simulink model "Experiment_Setup_Simulation"  (R2018b)
settings: Solver=FixedStepDiscrete  StartTime=0.0  StopTime=inf  FixedStep=0.02  RelTol=1e-3
libraries: simulink x4
settings Model: EnablePacing=on  PacingRate=2  Creator=Daniele Nava  LastModifiedBy=Daniele Nava

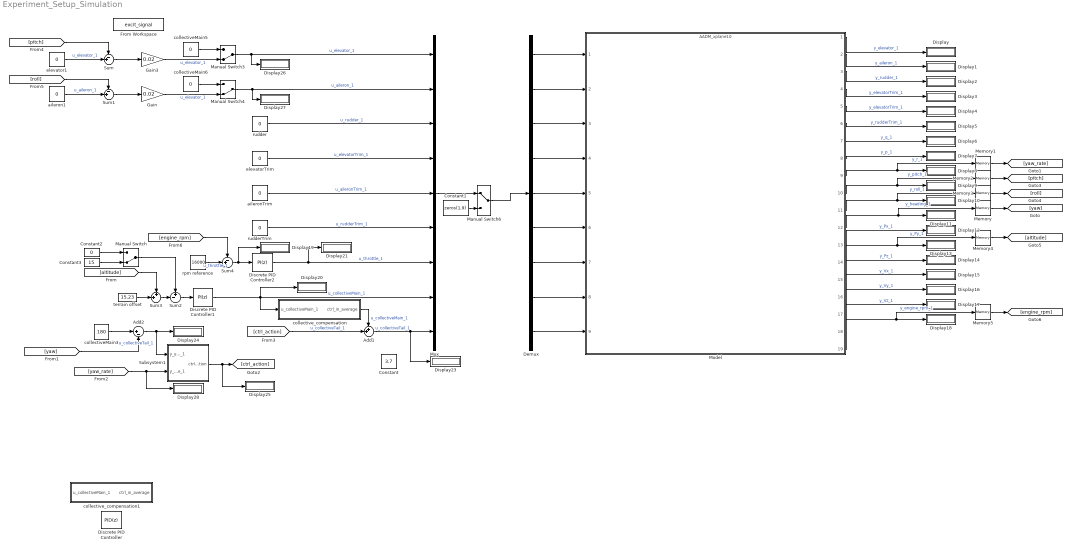
== system Experiment_Setup_Simulation ==
  Add1 : Sum  Inputs=++|
  Add2 : Sum  Inputs=|+-
  Constant : Constant  Value=3.7
  Constant1 : Constant  Value=zeros(1,9)
  Constant2 : Constant  Value=0
  Constant3 : Constant  Value=15
  Demux : Demux  Outputs=9
  Discrete PID Controller : simulink/Continuous/PID Controller  Controller=PID  Form=Parallel  TimeDomain=Discrete-time  SampleTime=-1  IntegratorMethod=Forward Euler  FilterMethod=Forward Euler  ControllerParametersSource=internal  P=1  I=1  D=0  UseFilter=on  N=100  TunerSelectOption=Transfer Function Based (PID Tuner App)  InitialConditionSource=internal  InitialConditionForIntegrator=0  InitialConditionForFilter=0  DifferentiatorICPrevScaledInput=0  ExternalReset=none  TrackingMode=off  Kt=1  LimitOutput=off  UpperSaturationLimit=inf  LowerSaturationLimit=-inf  LinearizeAsGain=off  AntiWindupMode=none  Kb=1  POutMin=[]  POutMax=[]  IOutMin=[]  IOutMax=[]  DOutMin=[]  DOutMax=[]  NOutMin=[]  NOutMax=[]  SumOutMin=[]  SumOutMax=[]  SaturationOutMin=[]  SaturationOutMax=[]  PParamMin=[]  PParamMax=[]  IParamMin=[]  IParamMax=[]  DParamMin=[]  DParamMax=[]  NParamMin=[]  NParamMax=[]  KbParamMin=[]  KbParamMax=[]  KtParamMin=[]  KtParamMax=[]  KbOutMin=[]  KbOutMax=[]  KtOutMin=[]  KtOutMax=[]  IntegratorOutMin=[]  IntegratorOutMax=[]  FilterOutMin=[]  FilterOutMax=[]  SumI1OutMin=[]  SumI1OutMax=[]  SumI2OutMin=[]  SumI2OutMax=[]  SumI3OutMin=[]  SumI3OutMax=[]  SumI4OutMin=[]  SumI4OutMax=[]  SumDOutMin=[]  SumDOutMax=[]  DifferentiatorOutMin=[]  DifferentiatorOutMax=[]  FilterDiffOutCoefMin=[]  FilterDiffOutCoefMax=[]  ReciprocalOutMin=[]  ReciprocalOutMax=[]  SumDenOutMin=[]  SumDenOutMax=[]  SumNumOutMin=[]  SumNumOutMax=[]  DivideOutMin=[]  DivideOutMax=[]  IntegratorContinuousStateAttributes=''  IntegratorStateMustResolveToSignalObject=off  IntegratorRTWStateStorageClass=Auto  FilterContinuousStateAttributes=''  FilterStateMustResolveToSignalObject=off  FilterRTWStateStorageClass=Auto  ParallelPVariant=InternalParameters  IdealPVariant=Disabled  IVariant=InternalParameters  DVariant=InternalParameters  IntegratorVariant=Discrete  SatVariant=Disabled  AWVariant=Passthrough  PCopyVariant=Disabled  TRVariant=Disabled  FdbkBlocksVariant=Forward  IdealPFdbkVariant=Disabled  SatFdbkVariant=Disabled  DerivativeFilterVariant=ForwardEulerFilter  NVariant=InternalParameters  NCopyVariant=Disabled  FilterICVariant=InternalICsFilter  IntegratorICVariant=InternalICs  ExternalResetVariant=Disabled  TRSumVariant=Passthrough  SumFdbkVariant=Disabled  SumVariant=Sum_PID
  Discrete PID Controller1 : simulink/Continuous/PID Controller  Controller=PI  Form=Parallel  TimeDomain=Discrete-time  SampleTime=-1  IntegratorMethod=Forward Euler  FilterMethod=Forward Euler  ControllerParametersSource=internal  P=0.5  I=0.2  D=0  UseFilter=on  N=100  TunerSelectOption=Transfer Function Based (PID Tuner App)  InitialConditionSource=internal  InitialConditionForIntegrator=0  InitialConditionForFilter=0  DifferentiatorICPrevScaledInput=0  ExternalReset=none  TrackingMode=off  Kt=1  LimitOutput=off  UpperSaturationLimit=inf  LowerSaturationLimit=-inf  LinearizeAsGain=off  AntiWindupMode=none  Kb=1  POutMin=[]  POutMax=[]  IOutMin=[]  IOutMax=[]  DOutMin=[]  DOutMax=[]  NOutMin=[]  NOutMax=[]  SumOutMin=[]  SumOutMax=[]  SaturationOutMin=[]  SaturationOutMax=[]  PParamMin=[]  PParamMax=[]  IParamMin=[]  IParamMax=[]  DParamMin=[]  DParamMax=[]  NParamMin=[]  NParamMax=[]  KbParamMin=[]  KbParamMax=[]  KtParamMin=[]  KtParamMax=[]  KbOutMin=[]  KbOutMax=[]  KtOutMin=[]  KtOutMax=[]  IntegratorOutMin=[]  IntegratorOutMax=[]  FilterOutMin=[]  FilterOutMax=[]  SumI1OutMin=[]  SumI1OutMax=[]  SumI2OutMin=[]  SumI2OutMax=[]  SumI3OutMin=[]  SumI3OutMax=[]  SumI4OutMin=[]  SumI4OutMax=[]  SumDOutMin=[]  SumDOutMax=[]  DifferentiatorOutMin=[]  DifferentiatorOutMax=[]  FilterDiffOutCoefMin=[]  FilterDiffOutCoefMax=[]  ReciprocalOutMin=[]  ReciprocalOutMax=[]  SumDenOutMin=[]  SumDenOutMax=[]  SumNumOutMin=[]  SumNumOutMax=[]  DivideOutMin=[]  DivideOutMax=[]  IntegratorContinuousStateAttributes=''  IntegratorStateMustResolveToSignalObject=off  IntegratorRTWStateStorageClass=Auto  FilterContinuousStateAttributes=''  FilterStateMustResolveToSignalObject=off  FilterRTWStateStorageClass=Auto  ParallelPVariant=InternalParameters  IdealPVariant=Disabled  IVariant=InternalParameters  DVariant=Disabled  IntegratorVariant=Discrete  SatVariant=Disabled  AWVariant=Passthrough  PCopyVariant=Disabled  TRVariant=Disabled  FdbkBlocksVariant=Forward  IdealPFdbkVariant=Disabled  SatFdbkVariant=Disabled  DerivativeFilterVariant=Disabled  NVariant=Disabled  NCopyVariant=Disabled_SignalSpec  FilterICVariant=Disabled  IntegratorICVariant=InternalICs  ExternalResetVariant=Disabled  TRSumVariant=Passthrough  SumFdbkVariant=Disabled  SumVariant=Sum_PI
  Discrete PID Controller2 : simulink/Continuous/PID Controller  Controller=PI  Form=Parallel  TimeDomain=Discrete-time  SampleTime=-1  IntegratorMethod=Forward Euler  FilterMethod=Forward Euler  ControllerParametersSource=internal  P=0.5  I=0.2  D=0  UseFilter=on  N=100  TunerSelectOption=Transfer Function Based (PID Tuner App)  InitialConditionSource=internal  InitialConditionForIntegrator=0  InitialConditionForFilter=0  DifferentiatorICPrevScaledInput=0  ExternalReset=none  TrackingMode=off  Kt=1  LimitOutput=off  UpperSaturationLimit=inf  LowerSaturationLimit=-inf  LinearizeAsGain=off  AntiWindupMode=none  Kb=1  POutMin=[]  POutMax=[]  IOutMin=[]  IOutMax=[]  DOutMin=[]  DOutMax=[]  NOutMin=[]  NOutMax=[]  SumOutMin=[]  SumOutMax=[]  SaturationOutMin=[]  SaturationOutMax=[]  PParamMin=[]  PParamMax=[]  IParamMin=[]  IParamMax=[]  DParamMin=[]  DParamMax=[]  NParamMin=[]  NParamMax=[]  KbParamMin=[]  KbParamMax=[]  KtParamMin=[]  KtParamMax=[]  KbOutMin=[]  KbOutMax=[]  KtOutMin=[]  KtOutMax=[]  IntegratorOutMin=[]  IntegratorOutMax=[]  FilterOutMin=[]  FilterOutMax=[]  SumI1OutMin=[]  SumI1OutMax=[]  SumI2OutMin=[]  SumI2OutMax=[]  SumI3OutMin=[]  SumI3OutMax=[]  SumI4OutMin=[]  SumI4OutMax=[]  SumDOutMin=[]  SumDOutMax=[]  DifferentiatorOutMin=[]  DifferentiatorOutMax=[]  FilterDiffOutCoefMin=[]  FilterDiffOutCoefMax=[]  ReciprocalOutMin=[]  ReciprocalOutMax=[]  SumDenOutMin=[]  SumDenOutMax=[]  SumNumOutMin=[]  SumNumOutMax=[]  DivideOutMin=[]  DivideOutMax=[]  IntegratorContinuousStateAttributes=''  IntegratorStateMustResolveToSignalObject=off  IntegratorRTWStateStorageClass=Auto  FilterContinuousStateAttributes=''  FilterStateMustResolveToSignalObject=off  FilterRTWStateStorageClass=Auto  ParallelPVariant=InternalParameters  IdealPVariant=Disabled  IVariant=InternalParameters  DVariant=Disabled  IntegratorVariant=Discrete  SatVariant=Disabled  AWVariant=Passthrough  PCopyVariant=Disabled  TRVariant=Disabled  FdbkBlocksVariant=Forward  IdealPFdbkVariant=Disabled  SatFdbkVariant=Disabled  DerivativeFilterVariant=Disabled  NVariant=Disabled  NCopyVariant=Disabled_SignalSpec  FilterICVariant=Disabled  IntegratorICVariant=InternalICs  ExternalResetVariant=Disabled  TRSumVariant=Passthrough  SumFdbkVariant=Disabled  SumVariant=Sum_PI
  Display{,1..21,23..28} (28 alike) : Display
  From Workspace : FromWorkspace  VariableName=excit_signal  SampleTime=0
  Gain : Gain  Gain=0.02
  Gain3 : Gain  Gain=0.02
  Manual Switch : ManualSwitch  CurrentSetting=0
  Manual Switch3 : ManualSwitch  CurrentSetting=0
  Manual Switch4 : ManualSwitch  CurrentSetting=0
  Manual Switch6 : ManualSwitch
  Memory{,1..5} (6 alike) : Memory
  Model : ModelReference  ModelNameDialog=AADM_xplane10.slx  SimulationMode=Normal  ModelReferenceVersion=1.12
  Mux : Mux  Inputs=9
  Subsystem1 : Subsystem  mask{Kp=-0.8, Ki=-0.01, Kd=+0.01}
      mask prompts: Kp "Proportional"; Ki "Integral"; Kd "Derivative"
  Sum : Sum  Inputs=-+|
  Sum1 : Sum  Inputs=-+|
  Sum2 : Sum  Inputs=+-|
  Sum3 : Sum  Inputs=++|
  Sum4 : Sum  Inputs=-+|
  aileron1 : Constant  Value=0
  aileronTrim : Constant  Value=0
  collectiveMain3 : Constant  Value=180
  collectiveMain5 : Constant  Value=0
  collectiveMain6 : Constant  Value=0
  collective_compensation : Subsystem
  collective_compensation1 : Subsystem
  elevator1 : Constant  Value=0
  elevatorTrim : Constant  Value=0
  rpm reference : Constant  Value=16000
  rudder : Constant  Value=0
  rudderTrim : Constant  Value=0
  terrain offset : Constant  Value=15.23
  wires:
  elevatorTrim/1 -> Mux/4  "u_elevatorTrim_1"
  Sum/1 -> Gain3/1
  Sum1/1 -> Gain/1
  aileronTrim/1 -> Mux/5  "u_aileronTrim_1"
  rudderTrim/1 -> Mux/6  "u_rudderTrim_1"
  Discrete PID Controller2/1 -> Display21/1, Mux/7  "u_throttle_1"
  Discrete PID Controller1/1 -> Display20/1, Mux/8, collective_compensation/1(u_collectiveMain_1)  "u_collectiveMain_1"
  rudder/1 -> Mux/3  "u_rudder_1"
  collectiveMain3/1 -> Add2/1
  Add2/1 -> Subsystem1/1(y_yaw_1), Display24/1  "u_collectiveTail_1"
  [ctrl_action] -> Add1/2  "u_collectiveTail_1"
  Add1/1 -> Display23/1, Mux/9  "u_collectiveTail_1"
  [yaw] -> Add2/2
  [yaw_rate] -> Display28/1, Subsystem1/2(y_yaw_rate_1)
  Subsystem1/1(ctrl_action) -> Display25/1, [ctrl_action]
  aileron1/1 -> Sum1/2  "u_aileron_1"
  elevator1/1 -> Sum/2  "u_elevator_1"
  [roll] -> Sum1/1
  [pitch] -> Sum/1
  Manual Switch3/1 -> Mux/1, Display26/1  "u_elevator_1"
  collectiveMain5/1 -> Manual Switch3/1
  Gain3/1 -> Manual Switch3/2  "u_elevator_1"
  Gain/1 -> Manual Switch4/2  "u_elevator_1"
  collectiveMain6/1 -> Manual Switch4/1
  Manual Switch4/1 -> Mux/2, Display27/1  "u_aileron_1"
  Memory3/1 -> [roll]
  Model/3 -> Display2/1  "y_rudder_1"
  Model/15 -> Display14/1  "y_Pz_1"
  Model/6 -> Display5/1  "y_rudderTrim_1"
  Memory2/1 -> [pitch]
  Model/2 -> Display1/1  "y_aileron_1"
  Model/8 -> Display7/1  "y_p_1"
  Model/4 -> Display3/1  "y_elevatorTrim_1"
  Model/10 -> Memory2/1, Display9/1  "y_pitch_1"
  Memory/1 -> [yaw]
  Model/1 -> Display/1  "y_elevator_1"
  Model/7 -> Display6/1  "y_q_1"
  Memory1/1 -> [yaw_rate]
  Model/17 -> Display16/1  "y_Vy_1"
  Model/12 -> Memory/1, Display11/1  "y_heading_1"
  Model/16 -> Display15/1  "y_Vx_1"
  Model/13 -> Display12/1  "y_Px_1"
  Model/11 -> Memory3/1, Display10/1  "y_roll_1"
  Model/18 -> Display17/1  "y_Vz_1"
  Model/5 -> Display4/1  "y_elevatorTrim_1"
  Model/9 -> Memory1/1, Display8/1  "y_r_1"
  Demux/1 -> Model/1
  Demux/2 -> Model/2
  Demux/3 -> Model/3
  Demux/4 -> Model/4
  Demux/5 -> Model/5
  Demux/6 -> Model/6
  Demux/7 -> Model/7
  Demux/8 -> Model/8
  Demux/9 -> Model/9
  Manual Switch6/1 -> Demux/1
  Mux/1 -> Manual Switch6/1
  Constant1/1 -> Manual Switch6/2
  Model/14 -> Memory4/1, Display13/1  "y_Py_1"
  Memory4/1 -> [altitude]
  Sum2/1 -> Discrete PID Controller1/1
  Sum3/1 -> Sum2/2
  Constant2/1 -> Manual Switch/1
  Constant3/1 -> Manual Switch/2
  terrain offset/1 -> Sum3/2
  [altitude] -> Sum3/1
  Manual Switch/1 -> Sum2/1
  Memory5/1 -> [engine_rpm]
  Model/19 -> Memory5/1, Display18/1  "y_engine_rpm_1"
  [engine_rpm] -> Sum4/1
  rpm reference/1 -> Sum4/2  "u_throttle_1"
  Sum4/1 -> Discrete PID Controller2/1, Display19/1
  collective_compensation/1(ctrl_in_average) -> Add1/1  "u_collectiveMain_1"

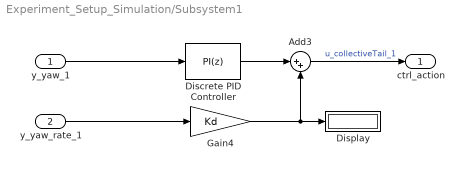
== system Experiment_Setup_Simulation/Subsystem1 ==
  y_yaw_1 : Inport
  y_yaw_rate_1 : Inport  Port=2
  Add3 : Sum  Inputs=|++
  Discrete PID Controller : simulink/Continuous/PID Controller  Controller=PI  Form=Parallel  TimeDomain=Discrete-time  SampleTime=-1  IntegratorMethod=Forward Euler  FilterMethod=Forward Euler  ControllerParametersSource=internal  P=Kp  I=Ki  D=0  UseFilter=on  N=100  TunerSelectOption=Transfer Function Based (PID Tuner App)  InitialConditionSource=internal  InitialConditionForIntegrator=0  InitialConditionForFilter=0  DifferentiatorICPrevScaledInput=0  ExternalReset=none  TrackingMode=off  Kt=1  LimitOutput=on  UpperSaturationLimit=16-8  LowerSaturationLimit=-16-8  LinearizeAsGain=off  AntiWindupMode=back-calculation  Kb=1  POutMin=[]  POutMax=[]  IOutMin=[]  IOutMax=[]  DOutMin=[]  DOutMax=[]  NOutMin=[]  NOutMax=[]  SumOutMin=[]  SumOutMax=[]  SaturationOutMin=[]  SaturationOutMax=[]  PParamMin=[]  PParamMax=[]  IParamMin=[]  IParamMax=[]  DParamMin=[]  DParamMax=[]  NParamMin=[]  NParamMax=[]  KbParamMin=[]  KbParamMax=[]  KtParamMin=[]  KtParamMax=[]  KbOutMin=[]  KbOutMax=[]  KtOutMin=[]  KtOutMax=[]  IntegratorOutMin=[]  IntegratorOutMax=[]  FilterOutMin=[]  FilterOutMax=[]  SumI1OutMin=[]  SumI1OutMax=[]  SumI2OutMin=[]  SumI2OutMax=[]  SumI3OutMin=[]  SumI3OutMax=[]  SumI4OutMin=[]  SumI4OutMax=[]  SumDOutMin=[]  SumDOutMax=[]  DifferentiatorOutMin=[]  DifferentiatorOutMax=[]  FilterDiffOutCoefMin=[]  FilterDiffOutCoefMax=[]  ReciprocalOutMin=[]  ReciprocalOutMax=[]  SumDenOutMin=[]  SumDenOutMax=[]  SumNumOutMin=[]  SumNumOutMax=[]  DivideOutMin=[]  DivideOutMax=[]  IntegratorContinuousStateAttributes=''  IntegratorStateMustResolveToSignalObject=off  IntegratorRTWStateStorageClass=Auto  FilterContinuousStateAttributes=''  FilterStateMustResolveToSignalObject=off  FilterRTWStateStorageClass=Auto  ParallelPVariant=InternalParameters  IdealPVariant=Disabled  IVariant=InternalParameters  DVariant=Disabled  IntegratorVariant=Discrete  SatVariant=Enabled  AWVariant=BackCalculation  PCopyVariant=Disabled  TRVariant=Disabled  FdbkBlocksVariant=Forward  IdealPFdbkVariant=Disabled  SatFdbkVariant=Disabled  DerivativeFilterVariant=Disabled  NVariant=Disabled  NCopyVariant=Disabled_SignalSpec  FilterICVariant=Disabled  IntegratorICVariant=InternalICs  ExternalResetVariant=Disabled  TRSumVariant=Passthrough  SumFdbkVariant=Disabled  SumVariant=Sum_PI
  Display : Display
  Gain4 : Gain  Gain=Kd
  ctrl_action : Outport
  wires:
  y_yaw_rate_1/1 -> Gain4/1
  Add3/1 -> ctrl_action/1  "u_collectiveTail_1"
  y_yaw_1/1 -> Discrete PID Controller/1
  Discrete PID Controller/1 -> Add3/1
  Gain4/1 -> Add3/2, Display/1

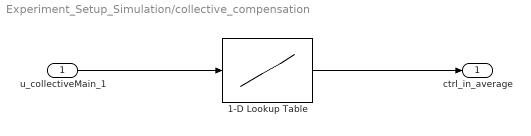
== system Experiment_Setup_Simulation/collective_compensation ==
  u_collectiveMain_1 : Inport
  1-D Lookup Table : Lookup_n-D  NumberOfTableDimensions=1  BreakpointsForDimension1=[-20,2.5,3,4,5,8,10,12,14,17, 20]  Table=[0, 0,3.7, 5.5, 7, 8.7, 11.5, 13.3, 15, 18, 18]  InternalRulePriority=Speed  RndMeth=Simplest  InputSameDT=on
  ctrl_in_average : Outport
  wires:
  u_collectiveMain_1/1 -> 1-D Lookup Table/1
  1-D Lookup Table/1 -> ctrl_in_average/1

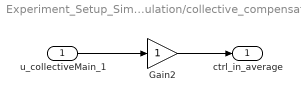
== system Experiment_Setup_Simulation/collective_compensation1 ==
  u_collectiveMain_1 : Inport
  Gain2 : Gain
  ctrl_in_average : Outport
  wires:
  Gain2/1 -> ctrl_in_average/1
  u_collectiveMain_1/1 -> Gain2/1
